simulink model "minmax_test"  (Simulink 9.0)
settings: Solver=FixedStepDiscrete  StartTime=0.0  StopTime=10.0  FixedStep=1.000000  RelTol=1e-3  EnableMultiTasking=on
settings Model: SuppressorTable=22 serialization::archive 11 0 6 0 0 0 0 0  Creator=arnaud  LastModifiedBy=hbourbou
settings DataIOCC: LimitDataPoints=on  SaveFormat=Structure  SignalLoggingSaveFormat=ModelDataLogs
settings OptimizationCC: ExpressionDepthLimit=2147483647
settings DebuggingCC: SolverPrmCheckMsg=warning  FcnCallInpInsideContextMsg=warning  StateNameClashWarn=warning  StrictBusMsg=Warning
settings GRTTargetCC: CombineOutputUpdateFcns=off  GRTInterface=on

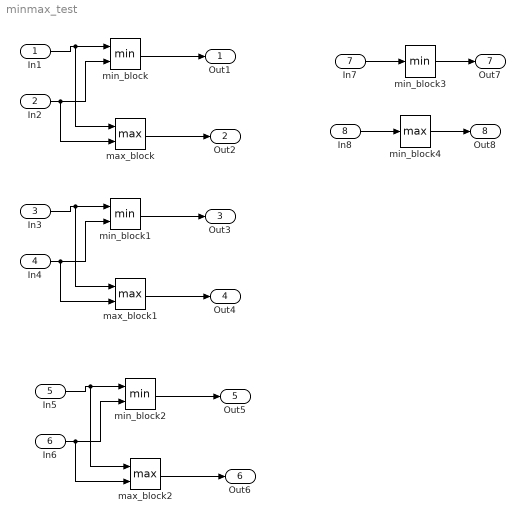
== system minmax_test ==
  In1 : Inport
  In2 : Inport  Port=2
  In3 : Inport  Port=3  PortDimensions=[2]
  In4 : Inport  Port=4  PortDimensions=[2]
  In5 : Inport  Port=5  PortDimensions=[2 2]
  In6 : Inport  Port=6  PortDimensions=[2 2]
  In7 : Inport  Port=7  PortDimensions=[3]
  In8 : Inport  Port=8  PortDimensions=[7]
  max_block : MinMax  Function=max  Inputs=2
  max_block1 : MinMax  Function=max  Inputs=2
  max_block2 : MinMax  Function=max  Inputs=2
  min_block : MinMax  Inputs=2
  min_block1 : MinMax  Inputs=2
  min_block2 : MinMax  Inputs=2
  min_block3 : MinMax
  min_block4 : MinMax  Function=max
  Out1 : Outport
  Out2 : Outport  Port=2
  Out3 : Outport  Port=3
  Out4 : Outport  Port=4
  Out5 : Outport  Port=5
  Out6 : Outport  Port=6
  Out7 : Outport  Port=7
  Out8 : Outport  Port=8
  wires:
  In1/1 -> min_block/1, max_block/1
  In2/1 -> min_block/2, max_block/2
  min_block/1 -> Out1/1
  max_block/1 -> Out2/1
  In3/1 -> min_block1/1, max_block1/1
  In4/1 -> min_block1/2, max_block1/2
  min_block1/1 -> Out3/1
  max_block1/1 -> Out4/1
  In5/1 -> min_block2/1, max_block2/1
  In6/1 -> min_block2/2, max_block2/2
  min_block2/1 -> Out5/1
  max_block2/1 -> Out6/1
  In7/1 -> min_block3/1
  min_block3/1 -> Out7/1
  In8/1 -> min_block4/1
  min_block4/1 -> Out8/1
